simulink model "task7c_damper_value_lessthan_1"  (R2024b)
settings: Solver=VariableStepAuto  StartTime=0.0  StopTime=10.0  RelTol=1e-3
values from neighbouring files (symbols this model uses):
  b = input("enter the value of damper constant (b):   ")    [damperEquMfile.m]    (also in damperEquMfile_b.m = 0)
  F = input("enter the value of force (F):  ")    [damperEquMfile.m]    (also in damperEquMfile_b.m = 1)
  k = input("enter the value of spring constant (K):   ")    [damperEquMfile.m]    (also in damperEquMfile_b.m = 20)
  M = input("enter the value of Mass (M):   ")    [damperEquMfile.m]    (also in damperEquMfile_b.m = 1)
settings Model: Creator=admin  LastModifiedBy=admin

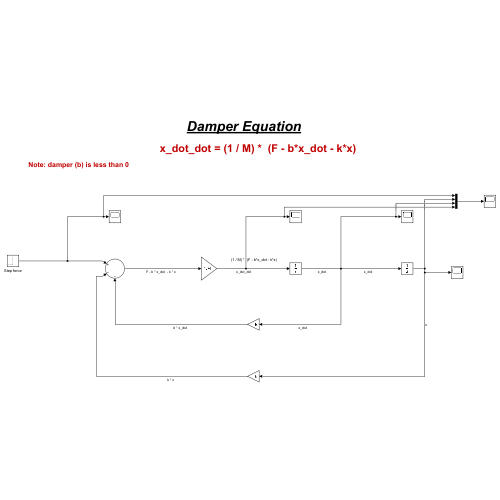
[thumbnail: Simulink's stored preview of the top-level diagram]
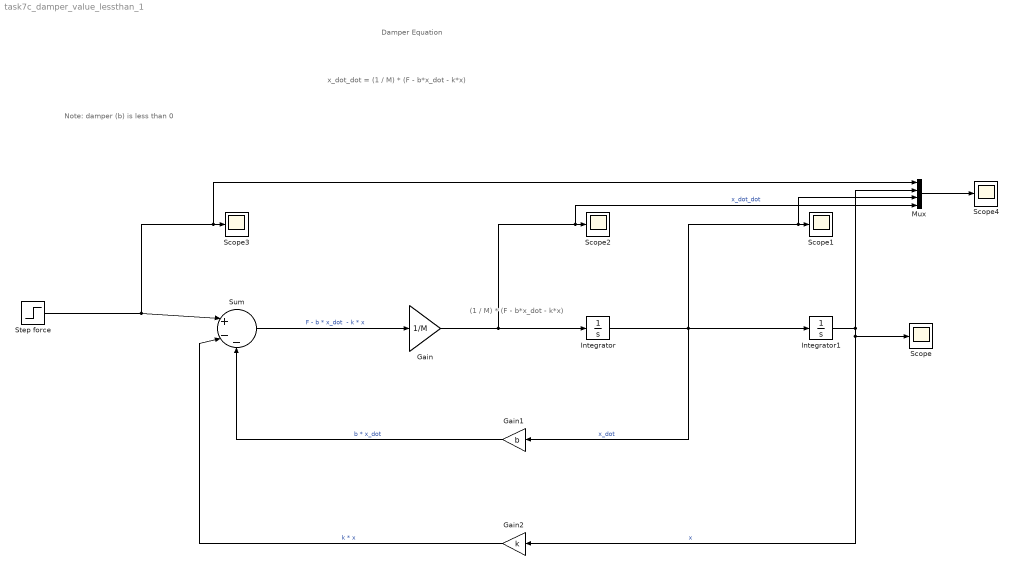
== system task7c_damper_value_lessthan_1 ==
  note: Note: damper (b) is less than 0
  note: Damper Equation
  note: (1 / M) * (F - b*x_dot - k*x)
  note: x_dot_dot = (1 / M) * (F - b*x_dot - k*x)
  Gain : Gain  Gain=1/M
  Gain1 : Gain  Gain=b
  Gain2 : Gain  Gain=k
  Integrator : Integrator
  Integrator1 : Integrator
  Mux : Mux
  Scope{,1..4} (5 alike) : Scope
  Step force : Step  After=F  SampleTime=0
  Sum : Sum  Inputs=|+--
  wires:
  Mux/1 -> Scope4/1
  Sum/1 -> Gain/1  "F - b * x_dot  - k * x"
  Integrator/1 -> Gain1/1, Mux/3, Scope1/1, Integrator1/1  "x_dot"
  Gain1/1 -> Sum/3  "b * x_dot"
  Gain2/1 -> Sum/2  "k * x"
  Integrator1/1 -> Gain2/1, Scope/1, Mux/2  "x"
  Gain/1 -> Mux/4, Scope2/1, Integrator/1  "x_dot_dot"
  Step force/1 -> Mux/1, Scope3/1, Sum/1
